simulink model "LAB1old"  (R2020b)
settings: Solver=ode45  StartTime=0.0  StopTime=10.0  MaxStep=0.01  RelTol=1e-3
values from neighbouring files (symbols this model uses):
  a1 = 6    [lab1.m]
  c1 = 4    [lab1.m]
  h10 = 0    [lab1.m]
  q10 = 5    [lab1.m]
settings Model: Creator=rfier  LastModifiedBy=Marek
settings OptimizationCC: LifeSpan=inf
settings DebuggingCC: ArithmeticOperatorsInVariantConditions=warning
settings SFSimCC: CustomCodeUndefinedFunction=UseInterfaceOnly
settings CodeAppCC: StateflowObjectComments=on

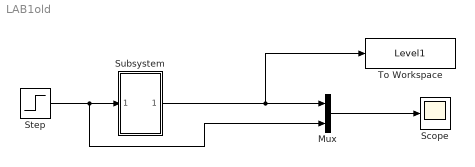
== system LAB1old ==
  Mux : Mux  Inputs=2
  Scope : Scope
  Step : Step  After=q10  SampleTime=0
  Subsystem : Subsystem
  To Workspace : ToWorkspace  VariableName=Level1  SampleTime=-1
  wires:
  Mux/1 -> Scope/1
  Step/1 -> Mux/2, Subsystem/1(In1)
  Subsystem/1(Out1) -> To Workspace/1, Mux/1

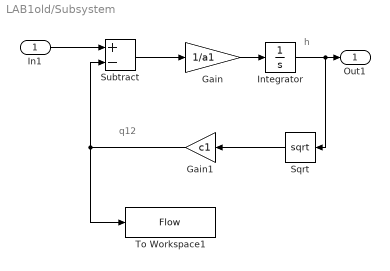
== system LAB1old/Subsystem ==
  note: h
  note: q12
  In1 : Inport
  Gain : Gain  Gain=1/a1
  Gain1 : Gain  Gain=c1
  Integrator : Integrator  InitialCondition=h10
  Sqrt : Sqrt  SaturateOnIntegerOverflow=on
  Subtract : Sum  Inputs=+-
  To Workspace1 : ToWorkspace  VariableName=Flow  SampleTime=-1
  Out1 : Outport
  wires:
  Gain/1 -> Integrator/1
  Gain1/1 -> To Workspace1/1, Subtract/2
  In1/1 -> Subtract/1
  Sqrt/1 -> Gain1/1
  Subtract/1 -> Gain/1
  Integrator/1 -> Sqrt/1, Out1/1
